simulink library "momentumVelocityControl_lib"  (R2019b)
settings: Solver=VariableStepAuto  StartTime=0.0  StopTime=10.0  RelTol=1e-3
undefined symbols (not defined in the file or in its folder): Gains, ROBOT_DOF, Sat, Weigth
libraries: WBToolboxLibrary x1
settings Model: Creator=csartore  LastModifiedBy=csartore

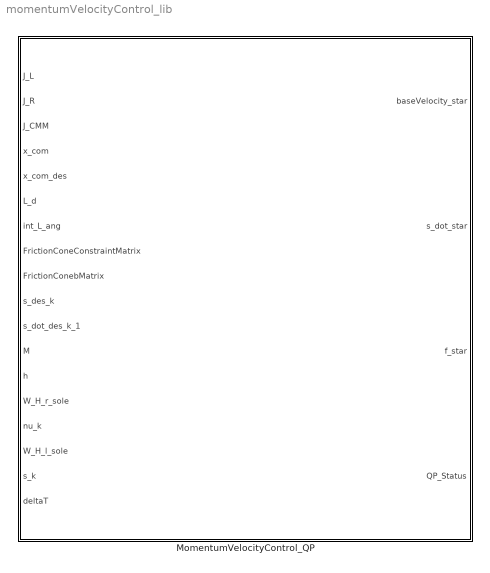
== system momentumVelocityControl_lib ==
  MomentumVelocityControl_QP : Subsystem

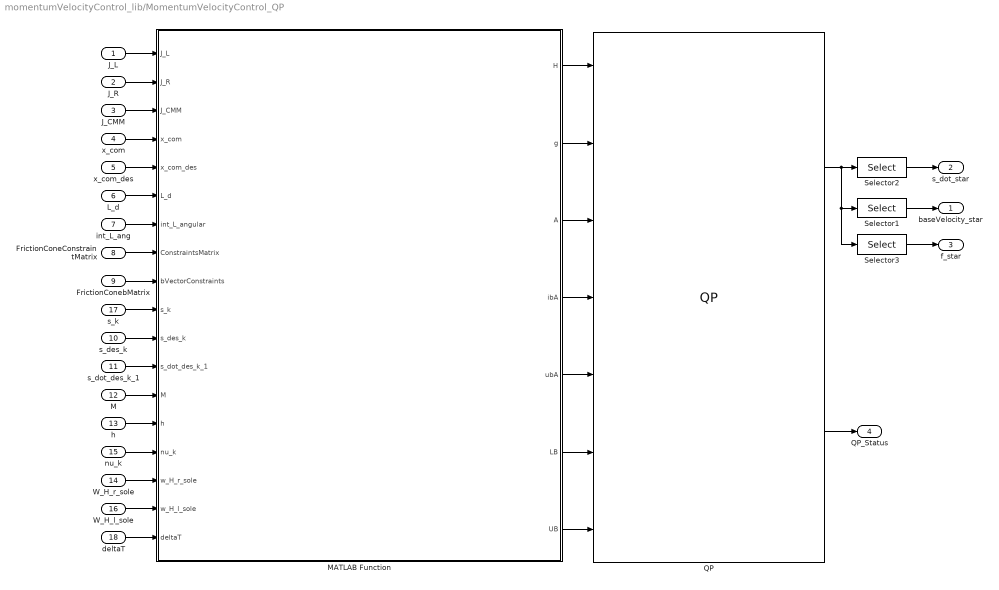
== system momentumVelocityControl_lib/MomentumVelocityControl_QP ==
  J_L : Inport
  J_R : Inport  Port=2
  J_CMM : Inport  Port=3
  x_com : Inport  Port=4
  x_com_des : Inport  Port=5
  L_d : Inport  Port=6
  int_L_ang : Inport  Port=7
  FrictionConeConstraintMatrix : Inport  Port=8
  FrictionConebMatrix : Inport  Port=9
  s_des_k : Inport  Port=10
  s_dot_des_k_1 : Inport  Port=11
  M : Inport  Port=12
  h : Inport  Port=13
  W_H_r_sole : Inport  Port=14
  nu_k : Inport  Port=15
  W_H_l_sole : Inport  Port=16
  s_k : Inport  Port=17
  "deltaT " : Inport  Port=18
  MATLAB Function : MATLAB Function  TreatAsAtomicUnit=on
  QP : WBToolboxLibrary/Utilities/QP  lbA=on  ubA=on  lb=on  ub=on  computeObjVal=off  stopIfFails=off
      settings: SourceProductName=WholeBodyToolbox
  Selector1 : Selector  InputPortWidth=18+ ROBOT_DOF  IndexOptions=Index vector (dialog)  Indices=[1:6]  OutputSizes=1
  Selector2 : Selector  InputPortWidth=18+ ROBOT_DOF  IndexOptions=Index vector (dialog)  Indices=[7:6+ROBOT_DOF]  OutputSizes=1
  Selector3 : Selector  InputPortWidth=18+ ROBOT_DOF  IndexOptions=Index vector (dialog)  Indices=[7+ ROBOT_DOF:18+ ROBOT_DOF]  OutputSizes=1
  baseVelocity_star : Outport
  s_dot_star : Outport  Port=2
  f_star : Outport  Port=3
  QP_Status : Outport  Port=4
  wires:
  QP/1 -> Selector3/1, Selector1/1, Selector2/1
  L_d/1 -> MATLAB Function/6(L_d)
  s_dot_des_k_1/1 -> MATLAB Function/12(s_dot_des_k_1)
  MATLAB Function/1(H) -> QP/1
  J_L/1 -> MATLAB Function/1(J_L)
  FrictionConeConstraintMatrix/1 -> MATLAB Function/8(ConstraintsMatrix)
  MATLAB Function/2(g) -> QP/2
  MATLAB Function/3(A) -> QP/3
  QP/2 -> QP_Status/1
  J_CMM/1 -> MATLAB Function/3(J_CMM)
  MATLAB Function/5(ubA) -> QP/5
  M/1 -> MATLAB Function/13(M)
  s_des_k/1 -> MATLAB Function/11(s_des_k)
  "deltaT "/1 -> MATLAB Function/18(deltaT)
  s_k/1 -> MATLAB Function/10(s_k)
  W_H_l_sole/1 -> MATLAB Function/17(w_H_l_sole)
  Selector1/1 -> baseVelocity_star/1
  nu_k/1 -> MATLAB Function/15(nu_k)
  FrictionConebMatrix/1 -> MATLAB Function/9(bVectorConstraints)
  W_H_r_sole/1 -> MATLAB Function/16(w_H_r_sole)
  J_R/1 -> MATLAB Function/2(J_R)
  x_com_des/1 -> MATLAB Function/5(x_com_des)
  MATLAB Function/6(LB) -> QP/6
  x_com/1 -> MATLAB Function/4(x_com)
  int_L_ang/1 -> MATLAB Function/7(int_L_angular)
  Selector2/1 -> s_dot_star/1
  MATLAB Function/7(UB) -> QP/7
  h/1 -> MATLAB Function/14(h)
  MATLAB Function/4(ibA) -> QP/4
  Selector3/1 -> f_star/1

== matlab function momentumVelocityControl_lib/MomentumVelocityControl_QP/MATLAB Function ==
  data: J_L input; H output; J_R input; J_CMM input; x_com input; x_com_des input; L_d input; int_L_angular input; ConstraintsMatrix input; bVectorConstraints input; s_k input; s_des_k input; s_dot_des_k_1 input; M input; h input; nu_k input; w_H_r_sole input; g output; A output; ibA output; ubA output; LB output; UB output; w_H_l_sole input; deltaT input; Gains parameter; Weigth parameter; Sat parameter
function [H, g, A, ibA, ubA, LB, UB] = MomentumVelocityControlFCN(J_L, J_R, J_CMM, x_com, x_com_des, L_d, int_L_angular, ...
    ConstraintsMatrix, bVectorConstraints,s_k,s_des_k, s_dot_des_k_1,M,h,nu_k,w_H_r_sole,w_H_l_sole,deltaT, Gains, Weigth, Sat)
[H, g, A, ibA, ubA, LB, UB] = MomentumVelocityControl(J_L, J_R, J_CMM, x_com, x_com_des, L_d, int_L_angular, ...
    ConstraintsMatrix, bVectorConstraints,s_k,s_des_k, s_dot_des_k_1,M,h,nu_k,w_H_r_sole,w_H_l_sole,deltaT, Gains,Weigth, Sat);
end
